simulink model "simulation"  (R2023b)
settings: Solver=VariableStepAuto  StartTime=0.0  StopTime=NN*N*h*CYCLES  RelTol=1e-3
InitFcn:
  | if ~exist('w_best')
  |     w_best = 0.9;
  | end
  | 
  | if ~exist('K')
  |     K = 1;
  | end
  | 
  | if ~exist('u_gain')
  |     u_gain = 1;
  | end
values from neighbouring files (symbols this model uses):
  h = 0.05    [main_bounds.m]    (also in run_dt_grad_ascent.m)
  N = 40    [main_bounds.m]    (also in main_gaussnewton.m = Nhorizon; run_dt_grad_ascent.m; run_generate_filters.m = MatrixPolynomial(Nb, order))
  NN = 10    [main.m]    (also in main_bounds.m; main_gaussnewton.m; main_ltv.m)
  NOISE = 1    [main.m]    (also in main_bounds.m; main_gaussnewton.m; main_ltv.m)
  R = tf(NL,tf('s'))/tf(den,1)    [run_generate_filters.m]
  simulink_seed = 22321    [main.m]    (also in main_bounds.m; main_gaussnewton.m = 22324; main_ltv.m)
  sys_fault = make_ss_from_dae(HF, LF)    [load_cart_pendulum_model.m]    (also in load_cart_pendulum_model_very_weak_motor.m)
  U = Ugood    [main.m]    (also in my_project.m = U*(length(u/m))^(1/type); run_dt_grad_ascent.m = reshape(u,m,[])')
libraries: simulink x6, cstblocks x4, dspinverses x1
settings Model: Creator=ggleizer  LastModifiedBy=ggleizer
settings ModelReferenceCC: EnableRefExpFcnMdlSchedulingChecks=on

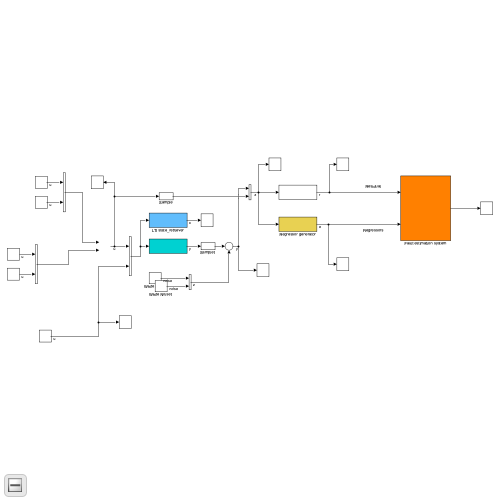
[thumbnail: Simulink's stored preview of the top-level diagram]
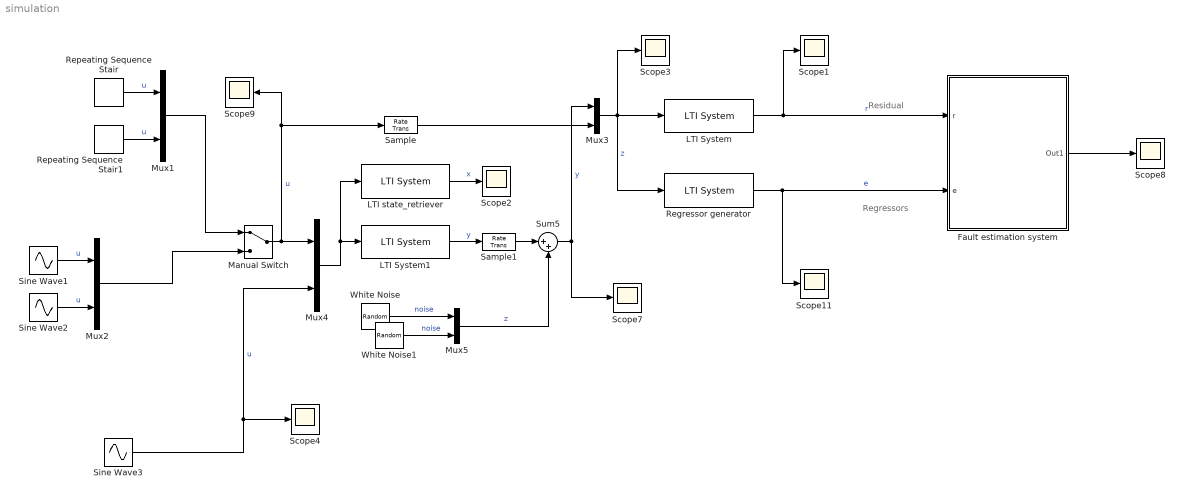
== system simulation ==
  note: Residual
  note: Regressors
  Fault estimation system : Subsystem
  LTI System : cstblocks/LTI System  sys=-R  IC=[]  PadeOrder=0
  LTI System1 : cstblocks/LTI System  sys=sys_fault  IC=[0.0; 0.0; 0.0]  PadeOrder=0
  LTI state_retriever : cstblocks/LTI System  sys=ss(sys_fault.A, sys_fault.B, eye(3), 0)  IC=[0.0; 0.0; 0.0]  PadeOrder=0
  Manual Switch : ManualSwitch
  Mux{1..5} (5 alike) : Mux  Inputs=2
  Regressor generator : cstblocks/LTI System  sys=Ms  IC=[0; 0.1; -1; 0]  PadeOrder=0
  Repeating Sequence Stair : simulink/Sources/Repeating Sequence Stair  OutValues=U(:,1)  tsamp=h  OutMin=[]  OutMax=[]  OutDataTypeStr=double  OutputDataTypeScalingMode=double  OutDataType=fixdt(0,8)  ConRadixGroup=Best Precision: Vector-wise  OutScaling=2^-12
  Repeating Sequence Stair1 : simulink/Sources/Repeating Sequence Stair  OutValues=U(:,2)  tsamp=h  OutMin=[]  OutMax=[]  OutDataTypeStr=double  OutputDataTypeScalingMode=double  OutDataType=fixdt(0,8)  ConRadixGroup=Best Precision: Vector-wise  OutScaling=2^-12
  Sample : RateTransition  OutPortSampleTime=0.02*h
  Sample1 : RateTransition  OutPortSampleTime=0.02*h
  Scope{1..4,7..9,11} (8 alike) : Scope
  Sine Wave1 : Sin  Frequency=2*pi/N/h  SampleTime=0
  Sine Wave2 : Sin  Frequency=2*pi/N/h  Phase=pi/2  SampleTime=0
  Sine Wave3 : Sin  Amplitude=5/180*pi  Frequency=pi  SampleTime=0
  Sum5 : Sum  Inputs=|++
  White Noise : RandomNumber  DisableCoverage=on  Variance=NOISE  Seed=simulink_seed  SampleTime=0.02*h
  White Noise1 : RandomNumber  DisableCoverage=on  Variance=NOISE  Seed=simulink_seed+1  SampleTime=0.02*h
  wires:
  Sum5/1 -> Mux3/1, Scope7/1  "y"
  LTI System1/1 -> Sample1/1  "y"
  Repeating Sequence Stair/1 -> Mux1/1  "u"
  Repeating Sequence Stair1/1 -> Mux1/2  "u"
  Mux1/1 -> Manual Switch/1
  Mux3/1 -> Scope3/1, LTI System/1, Regressor generator/1  "z"
  LTI System/1 -> Scope1/1, Fault estimation system/1(r)  "r"
  Regressor generator/1 -> Fault estimation system/2(e), Scope11/1  "e"
  Fault estimation system/1(Out1) -> Scope8/1
  Manual Switch/1 -> Mux4/1, Sample/1, Scope9/1  "u"
  Mux4/1 -> LTI state_retriever/1, LTI System1/1
  White Noise1/1 -> Mux5/2  "noise"
  White Noise/1 -> Mux5/1  "noise"
  Sine Wave2/1 -> Mux2/2  "u"
  Sine Wave1/1 -> Mux2/1  "u"
  Mux2/1 -> Manual Switch/2
  Sine Wave3/1 -> Scope4/1, Mux4/2  "u"
  Sample/1 -> Mux3/2
  Sample1/1 -> Sum5/1
  Mux5/1 -> Sum5/2  "z"
  LTI state_retriever/1 -> Scope2/1  "x"

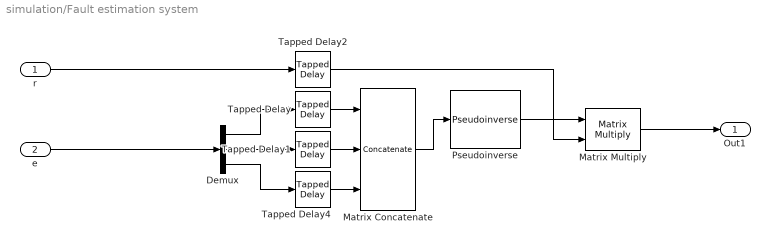
== system simulation/Fault estimation system ==
  r : Inport
  e : Inport  Port=2
  Demux : Demux  Outputs=3
  Matrix Concatenate : Concatenate  NumInputs=3  Mode=Multidimensional array  ConcatenateDimension=2
  Matrix Multiply : Product  Multiplication=Matrix(*)
  Pseudoinverse : dspinverses/Pseudoinverse  wanterr=off  SimulateUsing=Interpreted execution
  Tapped Delay{,1..2,4} (4 alike) : simulink/Discrete/Tapped Delay  vinit=0  samptime=h  NumDelays=N*NN  DelayOrder=Oldest  includeCurrent=on
  Out1 : Outport
  wires:
  Pseudoinverse/1 -> Matrix Multiply/1
  Tapped Delay4/1 -> Matrix Concatenate/3
  Tapped Delay1/1 -> Matrix Concatenate/2
  Tapped Delay2/1 -> Matrix Multiply/2
  Tapped Delay/1 -> Matrix Concatenate/1
  Matrix Multiply/1 -> Out1/1
  Demux/1 -> Tapped Delay/1
  Matrix Concatenate/1 -> Pseudoinverse/1
  e/1 -> Demux/1
  r/1 -> Tapped Delay2/1
  Demux/2 -> Tapped Delay1/1
  Demux/3 -> Tapped Delay4/1
